simulink model "Sist_completo_ensayo_temp_export"  (R2023b)
settings: Solver=VariableStepAuto  StartTime=0.0  StopTime=500  FixedStep=0.0001  MaxStep=6e-5  RelTol=1e-3
undefined symbols (not defined in the file): alpha_cu, b_a, b_eq, b_nom, C_ts, g, J_eq, J_nom, K_a, K_ai, k_l, k_l_nom, K_obs_theta, K_obs_w, L_d, L_ls, L_q, lambda_m, m_l, magnitude, P_p, r, R_0, R_d, R_q, R_sREF, R_ts_amb, T_amb, T_ld, T_sREF
libraries: SignalEditorBlockLib x2
settings Model: Creator=tomas  LastModifiedBy=tomas

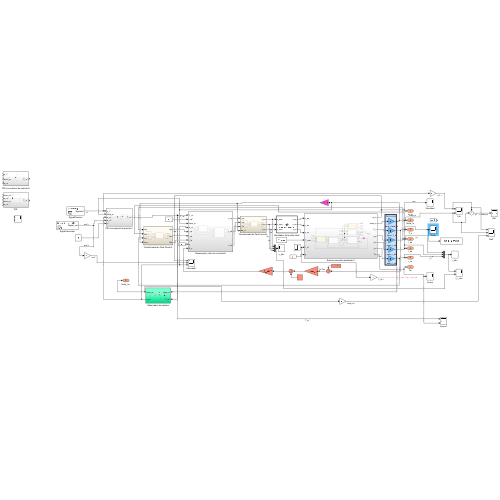
[thumbnail: Simulink's stored preview of the top-level diagram]
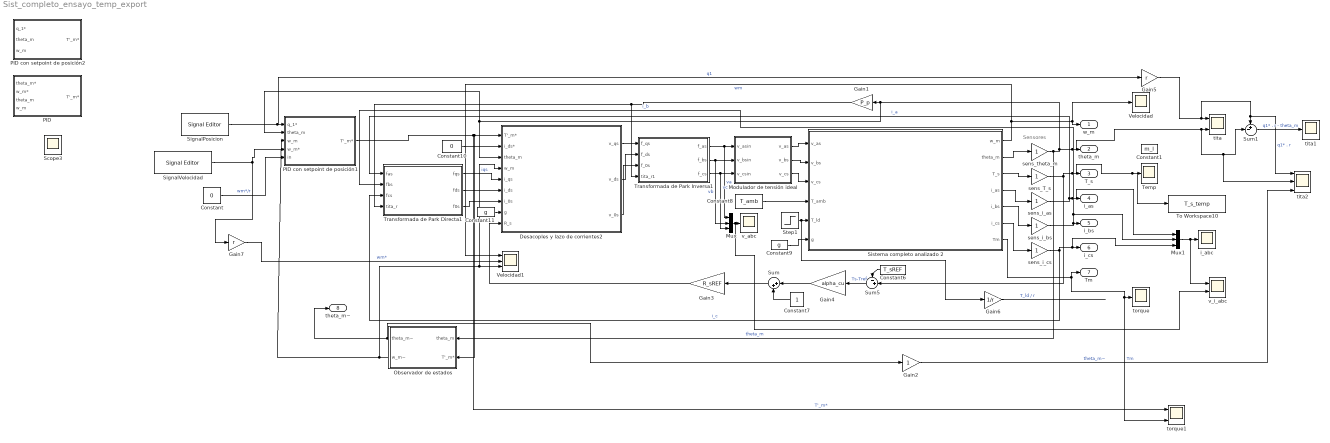
== system Sist_completo_ensayo_temp_export ==
  note: Sensores
  Constant : Constant  Value=0
  Constant1 : Constant  Value=m_l
  Constant10 : Constant  Value=0
  Constant11 : Constant  Value=g
  Constant6 : Constant  Value=T_sREF
  Constant7 : Constant
  Constant8 : Constant  Value=T_amb
  Constant9 : Constant  Value=g
  Desacoples y lazo de corrientes2 : Subsystem
  Gain1 : Gain  Gain=P_p
  Gain2 : Gain
  Gain3 : Gain  Gain=R_sREF
  Gain4 : Gain  Gain=alpha_cu
  Gain5 : Gain  Gain=r
  Gain6 : Gain  Gain=1/r
  Gain7 : Gain  Gain=r
  Modulador de tensión ideal : MATLAB Function  TreatAsAtomicUnit=on
  Mux : Mux  Inputs=3
  Mux1 : Mux  Inputs=3
  Observador de estados : Subsystem
  "PID " : Subsystem
  PID con setpoint de posición1 : Subsystem
  PID con setpoint de posición2 : Subsystem
  Scope3 : Scope  NumInputPorts=2
  SignalPosicion : SignalEditorBlockLib/Signal Editor  FileName=D:\Facu\Final AyME\Final-AyME\Simulink_LC\Simulacion\Signal\Perfil_trap_q1_25_veces.mat  ActiveScenario=Scenarioq1  ActiveSignal=Signalq1  IsBus=off  OutputBusObjectStr=Bus: BusObject  SampleTime=0  ZeroCross=off  OutputAfterFinalValue=Holding final value  Unit=inherit  PreserveSignalName=on  ApplySigPropsToAllScenarios=on  ApplySigPropsToAllSignals=off
  SignalVelocidad : SignalEditorBlockLib/Signal Editor  FileName=D:\Facu\Final AyME\Final-AyME\Simulink_LC\Simulacion\Signal\Perfil_trap_velocidad_25_veces.mat  ActiveScenario=Scenario_velocidad  ActiveSignal=Signal_vel  IsBus=off  OutputBusObjectStr=Bus: BusObject  SampleTime=0  ZeroCross=off  OutputAfterFinalValue=Holding final value  Unit=inherit  PreserveSignalName=on  ApplySigPropsToAllScenarios=on  ApplySigPropsToAllSignals=off
  Sistema completo analizado 2 : Subsystem
  Step1 : Step  Time=7.5  After=T_ld*0  SampleTime=0
  Sum : Sum  Inputs=|++
  Sum1 : Sum  Inputs=+-|
  Sum5 : Sum  Inputs=-+|
  Temp : Scope
  To Workspace10 : ToWorkspace  VariableName=T_s_temp  SaveFormat=Structure With Time  SampleTime=-1
  Transformada de Park Directa1 : Subsystem
  Transformada de Park Inversa1 : Subsystem
  Velocidad : Scope
  Velocidad1 : Scope  NumInputPorts=3
  i_abc : Scope
  sens_T_s : Gain
  sens_i_as : Gain
  sens_i_bs : Gain
  sens_i_cs : Gain
  sens_theta_m : Gain
  tita : Scope  NumInputPorts=2
  tita1 : Scope
  tita2 : Scope  NumInputPorts=3
  torque : Scope
  torque1 : Scope  NumInputPorts=2
  v_abc : Scope
  v_i_abc : Scope  NumInputPorts=2
  w_m : Outport
  theta_m : Outport  Port=2
  T_s : Outport  Port=3
  i_as : Outport  Port=4
  i_bs : Outport  Port=5
  i_cs : Outport  Port=6
  Tm : Outport  Port=7
  theta_m~ : Outport  Port=8
  wires:
  Sum5/1 -> Gain4/1  "Ts-Tref"
  Sistema completo analizado 2/5(i_bs) -> sens_i_bs/1
  sens_i_cs/1 -> Mux1/3, i_cs/1, Transformada de Park Directa1/3(fcs)  "i_c"
  Sistema completo analizado 2/4(i_as) -> sens_i_as/1
  Gain1/1 -> Transformada de Park Directa1/4(tita_r), Transformada de Park Inversa1/4(tita_r1)
  Modulador de tensión ideal/1(v_as) -> Sistema completo analizado 2/1(v_as)
  Transformada de Park Directa1/1(fqs) -> Desacoples y lazo de corrientes2/5(i_qs)  "iqs"
  Transformada de Park Directa1/2(fds) -> Desacoples y lazo de corrientes2/6(i_ds)
  Modulador de tensión ideal/2(v_bs) -> Sistema completo analizado 2/2(v_bs)
  Desacoples y lazo de corrientes2/2(v_ds) -> Transformada de Park Inversa1/2(f_ds)
  Transformada de Park Directa1/3(f0s) -> Desacoples y lazo de corrientes2/7(i_0s)
  Constant10/1 -> Desacoples y lazo de corrientes2/2(i_ds*)
  Constant8/1 -> Sistema completo analizado 2/4(T_amb)
  Sistema completo analizado 2/3(T_s) -> sens_T_s/1
  Transformada de Park Inversa1/1(f_as) -> Mux/1, Modulador de tensión ideal/1(v_asin)  "va"
  Desacoples y lazo de corrientes2/3(v_0s) -> Transformada de Park Inversa1/3(f_0s)
  Transformada de Park Inversa1/2(f_bs) -> Modulador de tensión ideal/2(v_bsin), Mux/2  "vb"
  PID con setpoint de posición1/1(T'_m*) -> Desacoples y lazo de corrientes2/1(T'_m*), Observador de estados/2(T'_m*), torque1/1  "T'_m*"
  Desacoples y lazo de corrientes2/1(v_qs) -> Transformada de Park Inversa1/1(f_qs)
  sens_T_s/1 -> Sum5/2, To Workspace10/1, Temp/1, T_s/1
  Transformada de Park Inversa1/3(f_cs) -> Modulador de tensión ideal/3(v_csin), Mux/3  "vc"
  Gain4/1 -> Sum/1
  Constant11/1 -> Desacoples y lazo de corrientes2/8(g)
  Constant7/1 -> Sum/2
  Modulador de tensión ideal/3(v_cs) -> Sistema completo analizado 2/3(v_cs)
  Constant6/1 -> Sum5/1
  Sum/1 -> Gain3/1
  Constant9/1 -> Sistema completo analizado 2/6(g)
  sens_i_bs/1 -> Transformada de Park Directa1/2(fbs), Mux1/2, i_bs/1  "i_b"
  sens_i_as/1 -> Transformada de Park Directa1/1(fas), Mux1/1, i_as/1  "i_a"
  Sistema completo analizado 2/2(theta_m) -> sens_theta_m/1
  Sistema completo analizado 2/6(i_cs) -> sens_i_cs/1
  Sistema completo analizado 2/7(Tm) -> torque1/2, torque/1, Tm/1  "Tm"
  Mux/1 -> v_i_abc/2, v_abc/1
  SignalPosicion/1 -> Gain5/1, PID con setpoint de posición1/1(q_1*)  "q1"
  Observador de estados/1(theta_m~) -> Gain2/1, theta_m~/1
  sens_theta_m/1 -> Observador de estados/1(theta_m), PID con setpoint de posición1/2(theta_m), Desacoples y lazo de corrientes2/3(theta_m), Gain1/1, tita2/2, Sum1/2, tita/2, theta_m/1  "theta_m"
  Step1/1 -> Gain6/1, Sistema completo analizado 2/5(T_ld)
  Sistema completo analizado 2/1(w_m) -> Velocidad1/1, w_m/1, Velocidad/1  "wm"
  Gain3/1 -> Desacoples y lazo de corrientes2/9(R_s)
  Gain5/1 -> tita2/1, Sum1/1, tita/1  "q1* . r"
  Sum1/1 -> tita1/1  "q1* . r - theta_m"
  Observador de estados/2(w_m~) -> PID con setpoint de posición1/3(w_m), Velocidad1/3, Desacoples y lazo de corrientes2/4(w_m)
  Mux1/1 -> v_i_abc/1, i_abc/1
  Gain2/1 -> tita2/3  "theta_m~"
  Gain6/1 -> ?  "T_ld / r"
  SignalVelocidad/1 -> PID con setpoint de posición1/4(w_m*), Gain7/1  "wm*/r"
  Constant/1 -> PID con setpoint de posición1/5(in)
  Gain7/1 -> Velocidad1/2  "wm*"

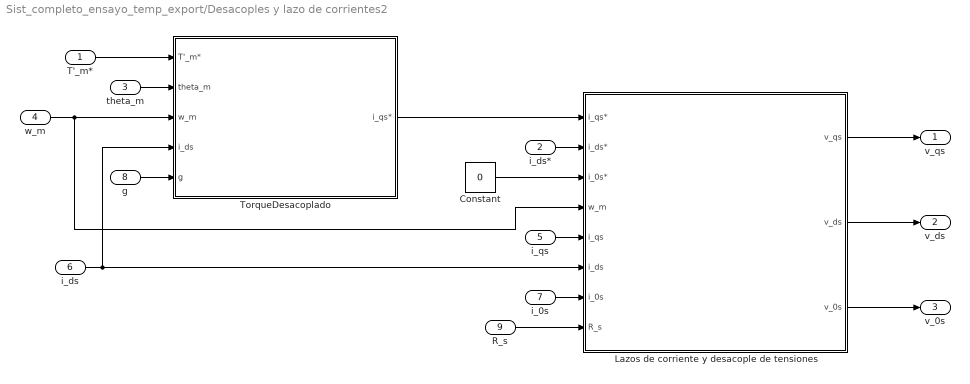
== system Sist_completo_ensayo_temp_export/Desacoples y lazo de corrientes2 ==
  T'_m* : Inport
  i_ds* : Inport  Port=2
  theta_m : Inport  Port=3
  w_m : Inport  Port=4
  i_qs : Inport  Port=5
  i_ds : Inport  Port=6
  i_0s : Inport  Port=7
  g : Inport  Port=8
  R_s : Inport  Port=9
  Constant : Constant  Value=0
  Lazos de corriente y desacople de tensiones : Subsystem
  TorqueDesacoplado : Subsystem
  v_qs : Outport
  v_ds : Outport  Port=2
  v_0s : Outport  Port=3
  wires:
  i_qs/1 -> Lazos de corriente y desacople de tensiones/5(i_qs)
  R_s/1 -> Lazos de corriente y desacople de tensiones/8(R_s)
  i_0s/1 -> Lazos de corriente y desacople de tensiones/7(i_0s)
  Constant/1 -> Lazos de corriente y desacople de tensiones/3(i_0s*)
  Lazos de corriente y desacople de tensiones/2(v_ds) -> v_ds/1
  Lazos de corriente y desacople de tensiones/1(v_qs) -> v_qs/1
  TorqueDesacoplado/1(i_qs*) -> Lazos de corriente y desacople de tensiones/1(i_qs*)
  Lazos de corriente y desacople de tensiones/3(v_0s) -> v_0s/1
  T'_m*/1 -> TorqueDesacoplado/1(T'_m*)
  theta_m/1 -> TorqueDesacoplado/2(theta_m)
  w_m/1 -> Lazos de corriente y desacople de tensiones/4(w_m), TorqueDesacoplado/3(w_m)
  i_ds/1 -> Lazos de corriente y desacople de tensiones/6(i_ds), TorqueDesacoplado/4(i_ds)
  g/1 -> TorqueDesacoplado/5(g)
  i_ds*/1 -> Lazos de corriente y desacople de tensiones/2(i_ds*)

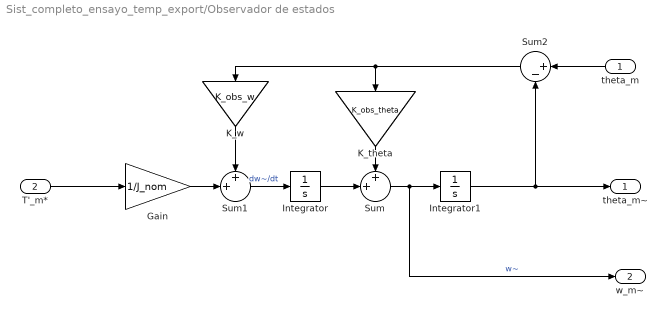
== system Sist_completo_ensayo_temp_export/Observador de estados ==
  theta_m : Inport
  T'_m* : Inport  Port=2
  Gain : Gain  Gain=1/J_nom
  Integrator : Integrator
  Integrator1 : Integrator
  K_theta : Gain  Gain=K_obs_theta
  K_w : Gain  Gain=K_obs_w
  Sum : Sum  Inputs=++|
  Sum1 : Sum  Inputs=++|
  Sum2 : Sum  Inputs=|+-
  theta_m~ : Outport
  w_m~ : Outport  Port=2
  wires:
  Gain/1 -> Sum1/2
  K_theta/1 -> Sum/1
  Sum1/1 -> Integrator/1  "dw~/dt"
  K_w/1 -> Sum1/1
  theta_m/1 -> Sum2/1
  Integrator/1 -> Sum/2
  Sum/1 -> w_m~/1, Integrator1/1  "w~"
  T'_m*/1 -> Gain/1
  Integrator1/1 -> theta_m~/1, Sum2/2
  Sum2/1 -> K_w/1, K_theta/1

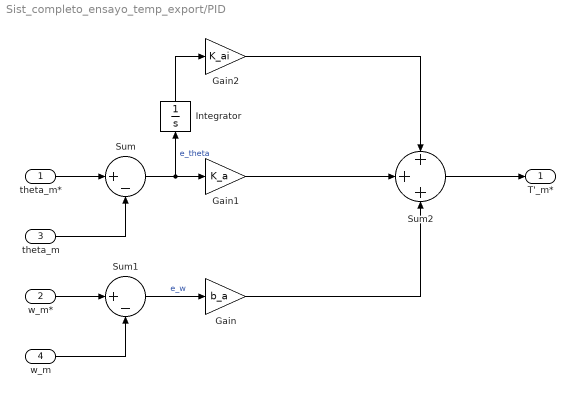
== system Sist_completo_ensayo_temp_export/PID  ==
  theta_m* : Inport
  w_m* : Inport  Port=2
  theta_m : Inport  Port=3
  w_m : Inport  Port=4
  Gain : Gain  Gain=b_a
  Gain1 : Gain  Gain=K_a
  Gain2 : Gain  Gain=K_ai
  Integrator : Integrator
  Sum : Sum  Inputs=|+-
  Sum1 : Sum  Inputs=|+-
  Sum2 : Sum  Inputs=+++
  T'_m* : Outport
  wires:
  Sum2/1 -> T'_m*/1
  Sum/1 -> Integrator/1, Gain1/1  "e_theta"
  Integrator/1 -> Gain2/1
  theta_m*/1 -> Sum/1
  Gain/1 -> Sum2/3
  Sum1/1 -> Gain/1  "e_w"
  w_m/1 -> Sum1/2
  Gain2/1 -> Sum2/1
  w_m*/1 -> Sum1/1
  Gain1/1 -> Sum2/2
  theta_m/1 -> Sum/2

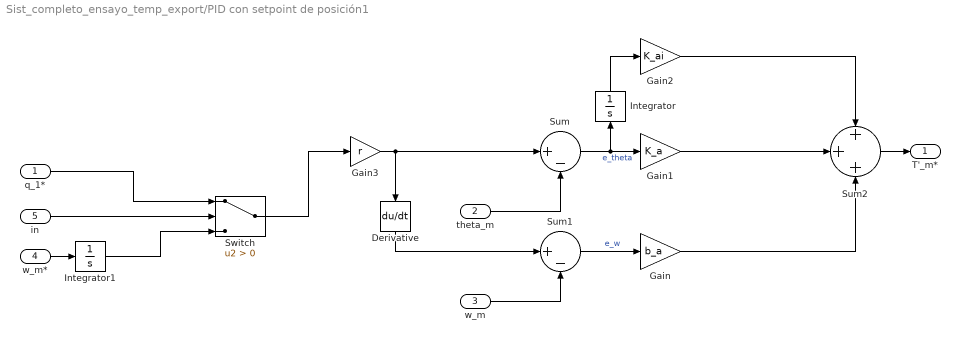
== system Sist_completo_ensayo_temp_export/PID con setpoint de posición1 ==
  q_1* : Inport
  theta_m : Inport  Port=2
  w_m : Inport  Port=3
  w_m* : Inport  Port=4
  in : Inport  Port=5
  Derivative : Derivative
  Gain : Gain  Gain=b_a
  Gain1 : Gain  Gain=K_a
  Gain2 : Gain  Gain=K_ai
  Gain3 : Gain  Gain=r
  Integrator : Integrator
  Integrator1 : Integrator
  Sum : Sum  Inputs=|+-
  Sum1 : Sum  Inputs=|+-
  Sum2 : Sum  Inputs=+++
  Switch : Switch  Criteria=u2 > Threshold  SaturateOnIntegerOverflow=off  InputSameDT=off
  T'_m* : Outport
  wires:
  Gain3/1 -> Sum/1, Derivative/1
  Derivative/1 -> Sum1/1
  Gain/1 -> Sum2/3
  Integrator/1 -> Gain2/1
  Sum2/1 -> T'_m*/1
  theta_m/1 -> Sum/2
  Gain1/1 -> Sum2/2
  Gain2/1 -> Sum2/1
  w_m/1 -> Sum1/2
  Sum/1 -> Integrator/1, Gain1/1  "e_theta"
  Sum1/1 -> Gain/1  "e_w"
  w_m*/1 -> Integrator1/1
  Switch/1 -> Gain3/1
  q_1*/1 -> Switch/1
  Integrator1/1 -> Switch/3
  in/1 -> Switch/2

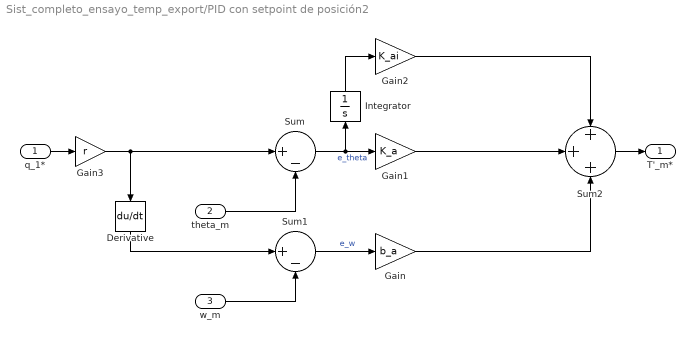
== system Sist_completo_ensayo_temp_export/PID con setpoint de posición2 ==
  q_1* : Inport
  theta_m : Inport  Port=2
  w_m : Inport  Port=3
  Derivative : Derivative
  Gain : Gain  Gain=b_a
  Gain1 : Gain  Gain=K_a
  Gain2 : Gain  Gain=K_ai
  Gain3 : Gain  Gain=r
  Integrator : Integrator
  Sum : Sum  Inputs=|+-
  Sum1 : Sum  Inputs=|+-
  Sum2 : Sum  Inputs=+++
  T'_m* : Outport
  wires:
  Gain3/1 -> Sum/1, Derivative/1
  Derivative/1 -> Sum1/1
  Gain/1 -> Sum2/3
  Integrator/1 -> Gain2/1
  q_1*/1 -> Gain3/1
  Sum2/1 -> T'_m*/1
  theta_m/1 -> Sum/2
  Gain1/1 -> Sum2/2
  Gain2/1 -> Sum2/1
  w_m/1 -> Sum1/2
  Sum/1 -> Integrator/1, Gain1/1  "e_theta"
  Sum1/1 -> Gain/1  "e_w"

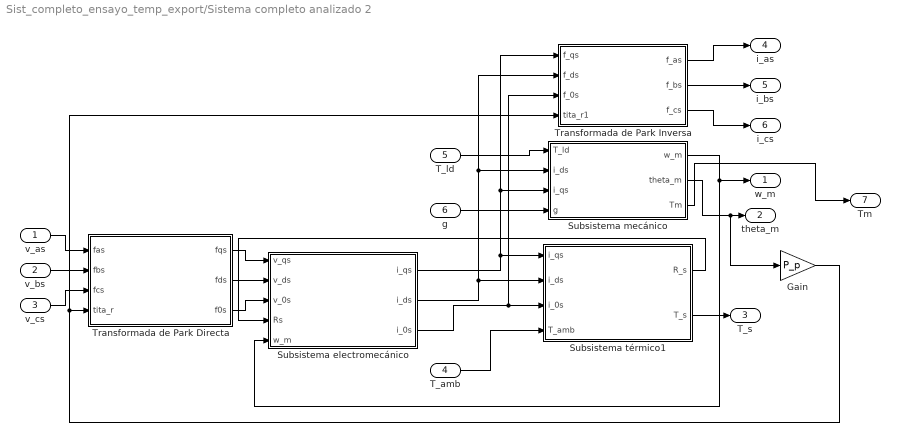
== system Sist_completo_ensayo_temp_export/Sistema completo analizado 2 ==
  v_as : Inport
  v_bs : Inport  Port=2
  v_cs : Inport  Port=3
  T_amb : Inport  Port=4
  T_ld : Inport  Port=5
  g : Inport  Port=6
  Gain : Gain  Gain=P_p
  Subsistema electromecánico : Subsystem
  Subsistema mecánico : Subsystem
  Subsistema térmico1 : Subsystem
  Transformada de Park Directa : Subsystem
  Transformada de Park Inversa : Subsystem
  w_m : Outport
  theta_m : Outport  Port=2
  T_s : Outport  Port=3
  i_as : Outport  Port=4
  i_bs : Outport  Port=5
  i_cs : Outport  Port=6
  Tm : Outport  Port=7
  wires:
  Transformada de Park Inversa/3(f_cs) -> i_cs/1
  Subsistema mecánico/1(w_m) -> w_m/1, Subsistema electromecánico/5(w_m)
  Subsistema electromecánico/3(i_0s) -> Subsistema térmico1/3(i_0s), Transformada de Park Inversa/3(f_0s)
  Transformada de Park Directa/1(fqs) -> Subsistema electromecánico/1(v_qs)
  Subsistema térmico1/2(T_s) -> T_s/1
  Transformada de Park Directa/3(f0s) -> Subsistema electromecánico/3(v_0s)
  Subsistema electromecánico/2(i_ds) -> Subsistema térmico1/2(i_ds), Transformada de Park Inversa/2(f_ds), Subsistema mecánico/2(i_ds)
  Gain/1 -> Transformada de Park Inversa/4(tita_r1), Transformada de Park Directa/4(tita_r)
  T_ld/1 -> Subsistema mecánico/1(T_ld)
  Transformada de Park Directa/2(fds) -> Subsistema electromecánico/2(v_ds)
  Transformada de Park Inversa/2(f_bs) -> i_bs/1
  v_bs/1 -> Transformada de Park Directa/2(fbs)
  T_amb/1 -> Subsistema térmico1/4(T_amb)
  Transformada de Park Inversa/1(f_as) -> i_as/1
  v_as/1 -> Transformada de Park Directa/1(fas)
  Subsistema mecánico/2(theta_m) -> Gain/1, theta_m/1
  v_cs/1 -> Transformada de Park Directa/3(fcs)
  Subsistema electromecánico/1(i_qs) -> Transformada de Park Inversa/1(f_qs), Subsistema mecánico/3(i_qs), Subsistema térmico1/1(i_qs)
  Subsistema térmico1/1(R_s) -> Subsistema electromecánico/4(Rs)
  g/1 -> Subsistema mecánico/4(g)
  Subsistema mecánico/3(Tm) -> Tm/1

== system Sist_completo_ensayo_temp_export/Transformada de Park Directa1 ==
  fas : Inport
  fbs : Inport  Port=2
  fcs : Inport  Port=3
  tita_r : Inport  Port=4
  MATLAB Function1 : MATLAB Function  TreatAsAtomicUnit=on
  fqs : Outport
  fds : Outport  Port=2
  f0s : Outport  Port=3
  wires:
  fas/1 -> MATLAB Function1/1(f_as)
  MATLAB Function1/3(f_0s) -> f0s/1
  MATLAB Function1/2(f_ds) -> fds/1
  fbs/1 -> MATLAB Function1/2(f_bs)
  fcs/1 -> MATLAB Function1/3(f_cs)
  tita_r/1 -> MATLAB Function1/4(tita_r)
  MATLAB Function1/1(f_qs) -> fqs/1

== system Sist_completo_ensayo_temp_export/Transformada de Park Inversa1 ==
  f_qs : Inport
  f_ds : Inport  Port=2
  f_0s : Inport  Port=3
  tita_r1 : Inport  Port=4
  MATLAB Function2 : MATLAB Function  TreatAsAtomicUnit=on
  f_as : Outport
  f_bs : Outport  Port=2
  f_cs : Outport  Port=3
  wires:
  tita_r1/1 -> MATLAB Function2/4(tita_r)
  MATLAB Function2/2(f_bs) -> f_bs/1
  MATLAB Function2/1(f_as) -> f_as/1
  f_ds/1 -> MATLAB Function2/2(f_ds)
  MATLAB Function2/3(f_cs) -> f_cs/1
  f_0s/1 -> MATLAB Function2/3(f_0s)
  f_qs/1 -> MATLAB Function2/1(f_qs)

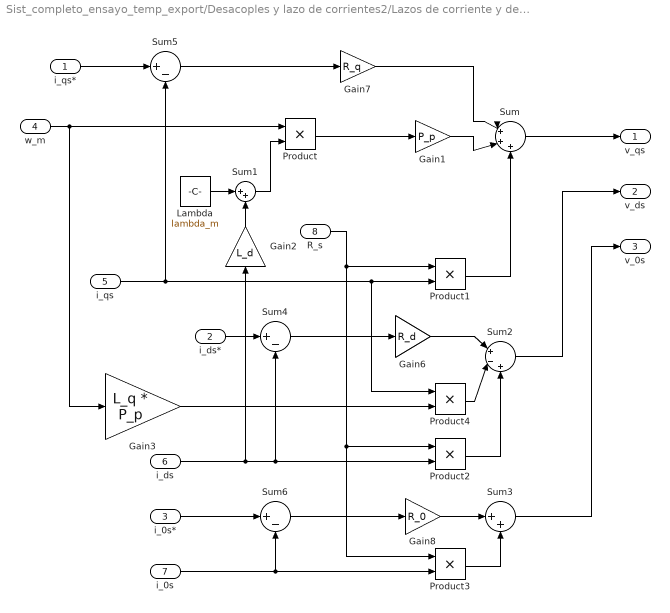
== system Sist_completo_ensayo_temp_export/Desacoples y lazo de corrientes2/Lazos de corriente y desacople de tensiones ==
  i_qs* : Inport
  i_ds* : Inport  Port=2
  i_0s* : Inport  Port=3
  w_m : Inport  Port=4
  i_qs : Inport  Port=5
  i_ds : Inport  Port=6
  i_0s : Inport  Port=7
  R_s : Inport  Port=8
  Gain1 : Gain  Gain=P_p
  Gain2 : Gain  Gain=L_d
  Gain3 : Gain  Gain=L_q * P_p
  Gain6 : Gain  Gain=R_d
  Gain7 : Gain  Gain=R_q
  Gain8 : Gain  Gain=R_0
  Lambda : Constant  Value=lambda_m
  Product{,1..4} (5 alike) : Product
  Sum : Sum  Inputs=|+++
  Sum1 : Sum  Inputs=|++
  Sum2 : Sum  Inputs=|+-+
  Sum3 : Sum  Inputs=|++
  Sum4 : Sum  Inputs=|+-
  Sum5 : Sum  Inputs=|+-
  Sum6 : Sum  Inputs=|+-
  v_qs : Outport
  v_ds : Outport  Port=2
  v_0s : Outport  Port=3
  wires:
  Product1/1 -> Sum/3
  Gain7/1 -> Sum/1
  R_s/1 -> Product3/1, Product2/1, Product1/1
  Sum6/1 -> Gain8/1
  Sum5/1 -> Gain7/1
  Gain8/1 -> Sum3/1
  Sum4/1 -> Gain6/1
  Gain3/1 -> Product4/2
  Gain6/1 -> Sum2/1
  i_ds*/1 -> Sum4/1
  Product2/1 -> Sum2/3
  i_0s*/1 -> Sum6/1
  Product3/1 -> Sum3/2
  i_0s/1 -> Product3/2, Sum6/2
  Sum2/1 -> v_ds/1
  Sum1/1 -> Product/2
  Gain1/1 -> Sum/2
  Sum/1 -> v_qs/1
  Product/1 -> Gain1/1
  Gain2/1 -> Sum1/2
  i_qs*/1 -> Sum5/1
  w_m/1 -> Gain3/1, Product/1
  Lambda/1 -> Sum1/1
  i_qs/1 -> Sum5/2, Product4/1, Product1/2
  Sum3/1 -> v_0s/1
  i_ds/1 -> Gain2/1, Product2/2, Sum4/2
  Product4/1 -> Sum2/2

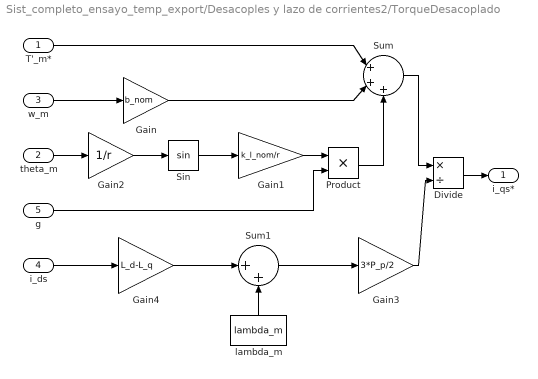
== system Sist_completo_ensayo_temp_export/Desacoples y lazo de corrientes2/TorqueDesacoplado ==
  T'_m* : Inport
  theta_m : Inport  Port=2
  w_m : Inport  Port=3
  i_ds : Inport  Port=4
  g : Inport  Port=5
  Divide : Product  Inputs=*/
  Gain : Gain  Gain=b_nom
  Gain1 : Gain  Gain=k_l_nom/r
  Gain2 : Gain  Gain=1/r
  Gain3 : Gain  Gain=3*P_p/2
  Gain4 : Gain  Gain=L_d-L_q
  Product : Product
  Sin : Trigonometry
  Sum : Sum  Inputs=|+++
  Sum1 : Sum  Inputs=|++
  lambda_m : Constant  Value=lambda_m
  i_qs* : Outport
  wires:
  T'_m*/1 -> Sum/1
  theta_m/1 -> Gain2/1
  Gain1/1 -> Product/1
  Sum1/1 -> Gain3/1
  Product/1 -> Sum/3
  i_ds/1 -> Gain4/1
  Divide/1 -> i_qs*/1
  Sin/1 -> Gain1/1
  Sum/1 -> Divide/1
  w_m/1 -> Gain/1
  lambda_m/1 -> Sum1/2
  Gain2/1 -> Sin/1
  Gain3/1 -> Divide/2
  Gain/1 -> Sum/2
  Gain4/1 -> Sum1/1
  g/1 -> Product/2

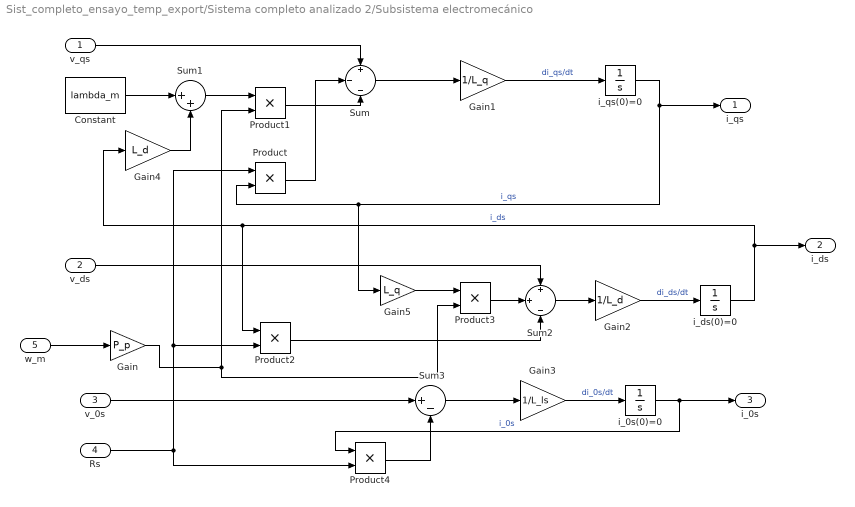
== system Sist_completo_ensayo_temp_export/Sistema completo analizado 2/Subsistema electromecánico ==
  v_qs : Inport
  v_ds : Inport  Port=2
  v_0s : Inport  Port=3
  Rs : Inport  Port=4
  w_m : Inport  Port=5
  Constant : Constant  Value=lambda_m
  Gain : Gain  Gain=P_p
  Gain1 : Gain  Gain=1/L_q
  Gain2 : Gain  Gain=1/L_d
  Gain3 : Gain  Gain=1/L_ls
  Gain4 : Gain  Gain=L_d
  Gain5 : Gain  Gain=L_q
  Product{,1..4} (5 alike) : Product
  Sum : Sum  Inputs=+|-|-
  Sum1 : Sum  Inputs=|++
  Sum2 : Sum  Inputs=+|+|-
  Sum3 : Sum  Inputs=|+-
  i_0s(0)=0 : Integrator
  i_ds(0)=0 : Integrator
  i_qs(0)=0 : Integrator
  i_qs : Outport
  i_ds : Outport  Port=2
  i_0s : Outport  Port=3
  wires:
  Gain1/1 -> i_qs(0)=0/1  "di_qs/dt"
  Rs/1 -> Product2/2, Product/1, Product4/2
  i_qs(0)=0/1 -> Gain5/1, Product/2, i_qs/1  "i_qs"
  Sum2/1 -> Gain2/1
  Product1/1 -> Sum/3
  Product4/1 -> Sum3/2
  v_0s/1 -> Sum3/1
  Product3/1 -> Sum2/2
  Gain3/1 -> i_0s(0)=0/1  "di_0s/dt"
  Gain/1 -> Product3/2, Product1/2
  v_qs/1 -> Sum/1
  Sum1/1 -> Product1/1
  Gain5/1 -> Product3/1
  Sum3/1 -> Gain3/1
  i_0s(0)=0/1 -> Product4/1, i_0s/1  "i_0s"
  Product2/1 -> Sum2/3
  Gain2/1 -> i_ds(0)=0/1  "di_ds/dt"
  Constant/1 -> Sum1/1
  Gain4/1 -> Sum1/2
  Sum/1 -> Gain1/1
  Product/1 -> Sum/2
  w_m/1 -> Gain/1
  i_ds(0)=0/1 -> Product2/1, Gain4/1, i_ds/1  "i_ds"
  v_ds/1 -> Sum2/1

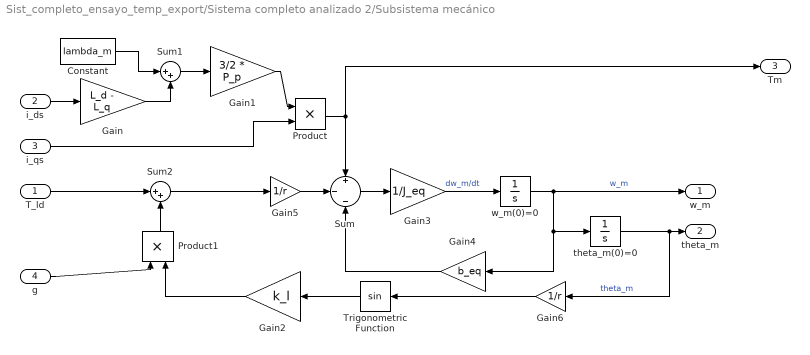
== system Sist_completo_ensayo_temp_export/Sistema completo analizado 2/Subsistema mecánico ==
  T_ld : Inport
  i_ds : Inport  Port=2
  i_qs : Inport  Port=3
  g : Inport  Port=4
  Constant : Constant  Value=lambda_m
  Gain : Gain  Gain=L_d - L_q
  Gain1 : Gain  Gain=3/2 * P_p
  Gain2 : Gain  Gain=k_l
  Gain3 : Gain  Gain=1/J_eq
  Gain4 : Gain  Gain=b_eq
  Gain5 : Gain  Gain=1/r
  Gain6 : Gain  Gain=1/r
  Product : Product
  Product1 : Product
  Sum : Sum  Inputs=+|-|-
  Sum1 : Sum  Inputs=|++
  Sum2 : Sum  Inputs=|++
  Trigonometric Function : Trigonometry
  theta_m(0)=0 : Integrator
  w_m(0)=0 : Integrator
  w_m : Outport
  theta_m : Outport  Port=2
  Tm : Outport  Port=3
  wires:
  w_m(0)=0/1 -> w_m/1, theta_m(0)=0/1, Gain4/1  "w_m"
  Sum/1 -> Gain3/1
  Gain3/1 -> w_m(0)=0/1  "dw_m/dt"
  i_ds/1 -> Gain/1
  Constant/1 -> Sum1/1
  Gain/1 -> Sum1/2
  Sum1/1 -> Gain1/1
  Gain1/1 -> Product/1
  i_qs/1 -> Product/2
  Gain4/1 -> Sum/3
  Gain5/1 -> Sum/2
  Trigonometric Function/1 -> Gain2/1
  Gain2/1 -> Product1/2
  theta_m(0)=0/1 -> Gain6/1, theta_m/1  "theta_m"
  T_ld/1 -> Sum2/1
  Sum2/1 -> Gain5/1
  Gain6/1 -> Trigonometric Function/1
  g/1 -> Product1/1
  Product1/1 -> Sum2/2
  Product/1 -> Sum/1, Tm/1

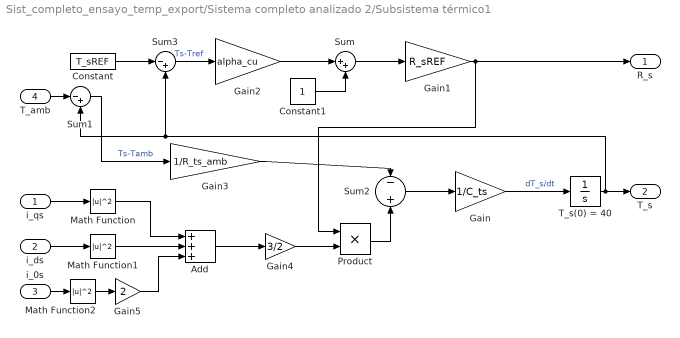
== system Sist_completo_ensayo_temp_export/Sistema completo analizado 2/Subsistema térmico1 ==
  i_qs : Inport
  i_ds : Inport  Port=2
  i_0s : Inport  Port=3
  T_amb : Inport  Port=4
  Add : Sum  Inputs=+++
  Constant : Constant  Value=T_sREF
  Constant1 : Constant
  Gain : Gain  Gain=1/C_ts
  Gain1 : Gain  Gain=R_sREF
  Gain2 : Gain  Gain=alpha_cu
  Gain3 : Gain  Gain=1/R_ts_amb
  Gain4 : Gain  Gain=3/2
  Gain5 : Gain  Gain=2
  Math Function : Math  Operator=magnitude^2
  Math Function1 : Math  Operator=magnitude^2
  Math Function2 : Math  Operator=magnitude^2
  Product : Product
  Sum : Sum  Inputs=|++
  Sum1 : Sum  Inputs=|-+
  Sum2 : Sum  Inputs=-|+
  Sum3 : Sum  Inputs=|-+
  T_s(0) = 40 : Integrator  InitialCondition=40
  R_s : Outport
  T_s : Outport  Port=2
  wires:
  Math Function2/1 -> Gain5/1
  Math Function/1 -> Add/1
  T_amb/1 -> Sum1/1
  Sum2/1 -> Gain/1
  Sum/1 -> Gain1/1
  Gain2/1 -> Sum/1
  Gain1/1 -> Product/1, R_s/1
  i_ds/1 -> Math Function1/1
  Gain/1 -> T_s(0) = 40/1  "dT_s/dt"
  Constant1/1 -> Sum/2
  Gain4/1 -> Product/2
  T_s(0) = 40/1 -> T_s/1, Sum3/2, Sum1/2
  Math Function1/1 -> Add/2
  i_0s/1 -> Math Function2/1
  Sum1/1 -> Gain3/1  "Ts-Tamb"
  Add/1 -> Gain4/1
  Gain5/1 -> Add/3
  i_qs/1 -> Math Function/1
  Gain3/1 -> Sum2/1
  Product/1 -> Sum2/2
  Constant/1 -> Sum3/1
  Sum3/1 -> Gain2/1  "Ts-Tref"

== system Sist_completo_ensayo_temp_export/Sistema completo analizado 2/Transformada de Park Directa ==
  fas : Inport
  fbs : Inport  Port=2
  fcs : Inport  Port=3
  tita_r : Inport  Port=4
  MATLAB Function1 : MATLAB Function  TreatAsAtomicUnit=on
  fqs : Outport
  fds : Outport  Port=2
  f0s : Outport  Port=3
  wires:
  fas/1 -> MATLAB Function1/1(f_as)
  MATLAB Function1/3(f_0s) -> f0s/1
  MATLAB Function1/2(f_ds) -> fds/1
  fbs/1 -> MATLAB Function1/2(f_bs)
  fcs/1 -> MATLAB Function1/3(f_cs)
  tita_r/1 -> MATLAB Function1/4(tita_r)
  MATLAB Function1/1(f_qs) -> fqs/1

== system Sist_completo_ensayo_temp_export/Sistema completo analizado 2/Transformada de Park Inversa ==
  f_qs : Inport
  f_ds : Inport  Port=2
  f_0s : Inport  Port=3
  tita_r1 : Inport  Port=4
  MATLAB Function2 : MATLAB Function  TreatAsAtomicUnit=on
  f_as : Outport
  f_bs : Outport  Port=2
  f_cs : Outport  Port=3
  wires:
  tita_r1/1 -> MATLAB Function2/4(tita_r)
  MATLAB Function2/2(f_bs) -> f_bs/1
  MATLAB Function2/1(f_as) -> f_as/1
  f_ds/1 -> MATLAB Function2/2(f_ds)
  MATLAB Function2/3(f_cs) -> f_cs/1
  f_0s/1 -> MATLAB Function2/3(f_0s)
  f_qs/1 -> MATLAB Function2/1(f_qs)

== matlab function Sist_completo_ensayo_temp_export/Transformada de Park Inversa1/MATLAB Function2 ==
  data: f_qs input; f_as output; f_ds input; f_0s input; tita_r input; f_bs output; f_cs output
function [f_as, f_bs, f_cs] = parkInv(f_qs,f_ds,f_0s,tita_r)

answer = [cos(tita_r), sin(tita_r), 1;
         cos(tita_r - 2*pi/3), sin(tita_r - 2*pi/3), 1;
         cos(tita_r + 2*pi/3), sin(tita_r + 2*pi/3), 1] * [f_qs;f_ds;f_0s]; 

f_as = answer(1);
f_bs = answer(2);
f_cs = answer(3);

== matlab function Sist_completo_ensayo_temp_export/Modulador de tensión ideal ==
  data: v_asin input; v_as output; v_bsin input; v_csin input; v_bs output; v_cs output
function [v_as,v_bs,v_cs] = ModuladorIdeal(v_asin,v_bsin, v_csin)
v_as=v_asin;
v_bs=v_bsin;
v_cs=v_csin;

== matlab function Sist_completo_ensayo_temp_export/Sistema completo analizado 2/Transformada de Park Directa/MATLAB Function1 ==
  data: f_as input; f_qs output; f_bs input; f_cs input; tita_r input; f_ds output; f_0s output
function [f_qs, f_ds, f_0s] = parkDir(f_as,f_bs,f_cs,tita_r)

answer = 2/3 * [cos(tita_r), cos(tita_r - 2*pi/3), cos(tita_r + 2*pi/3);
         sin(tita_r), sin(tita_r - 2*pi/3), sin(tita_r + 2*pi/3);
         1/2, 1/2, 1/2] * [f_as;f_bs;f_cs];

f_qs = answer(1);
f_ds = answer(2);
f_0s = answer(3);

== matlab function Sist_completo_ensayo_temp_export/Sistema completo analizado 2/Transformada de Park Inversa/MATLAB Function2 ==
  data: f_qs input; f_as output; f_ds input; f_0s input; tita_r input; f_bs output; f_cs output
function [f_as, f_bs, f_cs] = parkInv(f_qs,f_ds,f_0s,tita_r)

answer = [cos(tita_r), sin(tita_r), 1;
         cos(tita_r - 2*pi/3), sin(tita_r - 2*pi/3), 1;
         cos(tita_r + 2*pi/3), sin(tita_r + 2*pi/3), 1] * [f_qs;f_ds;f_0s]; 

f_as = answer(1);
f_bs = answer(2);
f_cs = answer(3);

== matlab function Sist_completo_ensayo_temp_export/Transformada de Park Directa1/MATLAB Function1 ==
  data: f_as input; f_qs output; f_bs input; f_cs input; tita_r input; f_ds output; f_0s output
function [f_qs, f_ds, f_0s] = parkDir(f_as,f_bs,f_cs,tita_r)

answer = 2/3 * [cos(tita_r), cos(tita_r - 2*pi/3), cos(tita_r + 2*pi/3);
         sin(tita_r), sin(tita_r - 2*pi/3), sin(tita_r + 2*pi/3);
         1/2, 1/2, 1/2] * [f_as;f_bs;f_cs];

f_qs = answer(1);
f_ds = answer(2);
f_0s = answer(3);
